simulink model "as5_filtering"  (R2019a)
settings: Solver=VariableStepAuto  StartTime=0.0  StopTime=50  MaxStep=0.01  RelTol=1e-3
settings Model: Creator=revolt  LastModifiedBy=revolt

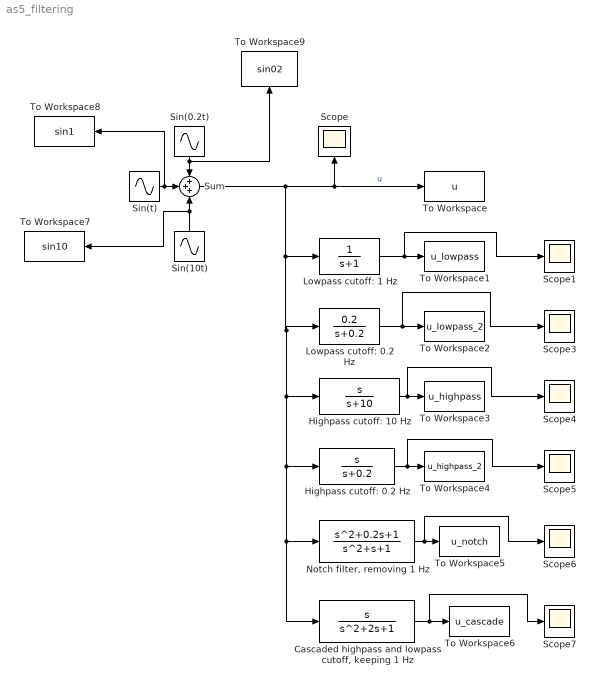
== system as5_filtering ==
  "Cascaded highpass and lowpass cutoff, keeping 1 Hz" : TransferFcn  Numerator=[1 0]
  Highpass cutoff: 0.2 Hz : TransferFcn  Numerator=[1 0]  Denominator=[1 0.2]
  Highpass cutoff: 10 Hz : TransferFcn  Numerator=[1 0]  Denominator=[1 10]
  Lowpass cutoff: 0.2 Hz : TransferFcn  Numerator=[0.2]  Denominator=[1 0.2]
  Lowpass cutoff: 1 Hz : TransferFcn  Denominator=[1 1]
  "Notch filter, removing 1 Hz" : TransferFcn  Numerator=[1 0.2 1]  Denominator=[1 1 1]
  Scope{,1,3..7} (7 alike) : Scope
  Sin(0.2t) : Sin  Frequency=0.2  SampleTime=0
  Sin(10t) : Sin  Frequency=10  SampleTime=0
  Sin(t) : Sin  SampleTime=0
  Sum : Sum  Inputs=+++
  To Workspace : ToWorkspace  VariableName=u  SaveFormat=Timeseries  SampleTime=-1
  To Workspace1 : ToWorkspace  VariableName=u_lowpass  SaveFormat=Timeseries  SampleTime=-1
  To Workspace2 : ToWorkspace  VariableName=u_lowpass_2  SaveFormat=Timeseries  SampleTime=-1
  To Workspace3 : ToWorkspace  VariableName=u_highpass  SaveFormat=Timeseries  SampleTime=-1
  To Workspace4 : ToWorkspace  VariableName=u_highpass_2  SaveFormat=Timeseries  SampleTime=-1
  To Workspace5 : ToWorkspace  VariableName=u_notch  SaveFormat=Timeseries  SampleTime=-1
  To Workspace6 : ToWorkspace  VariableName=u_cascade  SaveFormat=Timeseries  SampleTime=-1
  To Workspace7 : ToWorkspace  VariableName=sin10  SaveFormat=Timeseries  SampleTime=-1
  To Workspace8 : ToWorkspace  VariableName=sin1  SaveFormat=Timeseries  SampleTime=-1
  To Workspace9 : ToWorkspace  VariableName=sin02  SaveFormat=Timeseries  SampleTime=-1
  wires:
  Sin(t)/1 -> To Workspace8/1, Sum/2
  Sin(0.2t)/1 -> To Workspace9/1, Sum/1
  Sin(10t)/1 -> To Workspace7/1, Sum/3
  Sum/1 -> Scope/1, To Workspace/1, "Cascaded highpass and lowpass cutoff, keeping 1 Hz"/1, "Notch filter, removing 1 Hz"/1, Highpass cutoff: 0.2 Hz/1, Highpass cutoff: 10 Hz/1, Lowpass cutoff: 0.2 Hz/1, Lowpass cutoff: 1 Hz/1  "u"
  Lowpass cutoff: 1 Hz/1 -> Scope1/1, To Workspace1/1
  Lowpass cutoff: 0.2 Hz/1 -> Scope3/1, To Workspace2/1
  Highpass cutoff: 10 Hz/1 -> Scope4/1, To Workspace3/1
  Highpass cutoff: 0.2 Hz/1 -> Scope5/1, To Workspace4/1
  "Notch filter, removing 1 Hz"/1 -> Scope6/1, To Workspace5/1
  "Cascaded highpass and lowpass cutoff, keeping 1 Hz"/1 -> Scope7/1, To Workspace6/1
